simulink model "ARO40506DOF_2020a_2025_LAT"  (R2025b)
settings: Solver=VariableStepAuto  StartTime=0.0  StopTime=10.0  RelTol=1e-3
values from neighbouring files (symbols this model uses):
  Clbeta = -0.095    [Sim6DOF_Init.m]
  CldA = 0.014    [Sim6DOF_Init.m]
  CldR = 0.005    [Sim6DOF_Init.m]
  Cnbeta = 0.210    (= 0.21)    [Sim6DOF_Init.m]
  CndA = -0.0028    [Sim6DOF_Init.m]
  CndR = -0.095    [Sim6DOF_Init.m]
  Cybeta = -0.90    (= -0.9)    [Sim6DOF_Init.m]
  CydA = 0.0    (= 0)    [Sim6DOF_Init.m]
  CydR = 0.60    (= 0.6)    [Sim6DOF_Init.m]
  D2R = pi/180    (= 0.0174532925199)    [Sim6DOF_Init.m]
  q0 = 0    [Sim6DOF_Init.m]
  Span = 212.5    [Sim6DOF_Init.m]
  Sref = 4702    [Sim6DOF_Init.m]
  StabTrimPos = 5.5    [Sim6DOF_Init.m]
undefined symbols (not defined in the file or in its folder): Q
libraries: aerolibactuator x2
settings Model: Creator=Rainman  LastModifiedBy=Jordan Baylos
settings SolverCC: AlgebraicLoopSolver=TrustRegion
settings RTWCC: GPUComputeCapability=3.5

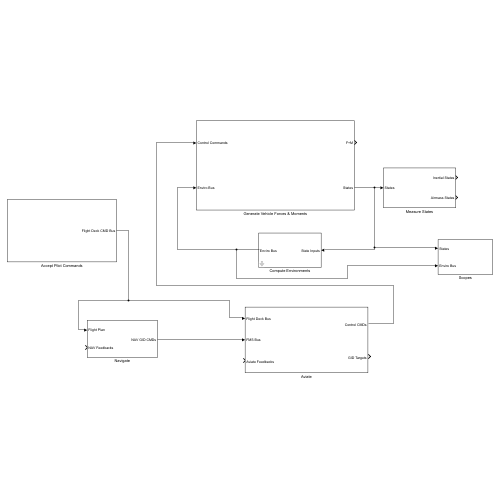
[thumbnail: Simulink's stored preview of the top-level diagram]
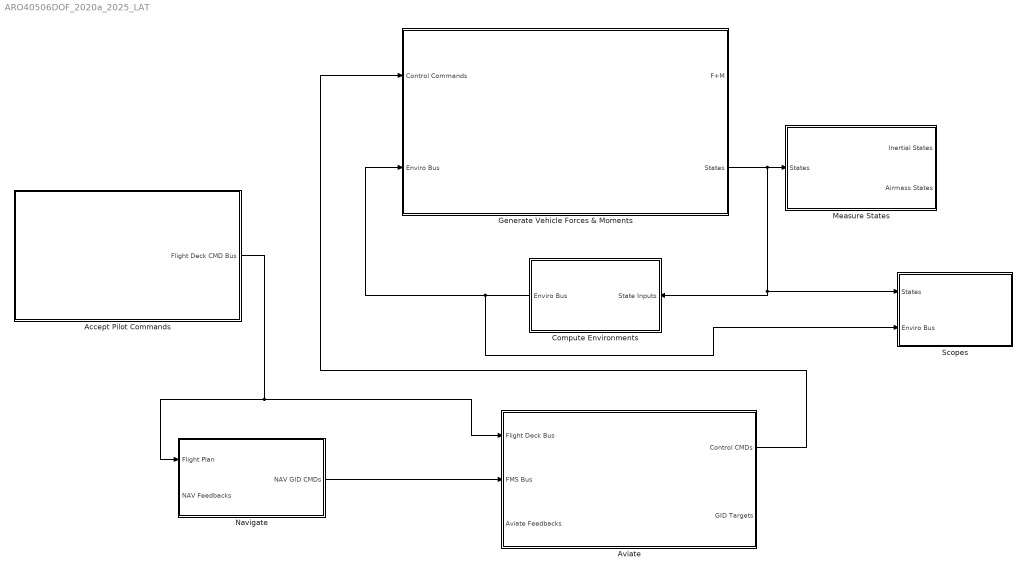
== system ARO40506DOF_2020a_2025_LAT ==
  Accept Pilot Commands : Subsystem
  Aviate : Subsystem
  Compute Environments : Subsystem
  Generate Vehicle Forces & Moments : Subsystem
  Measure States : Subsystem
  Navigate : Subsystem
  Scopes : Subsystem
  wires:
  Navigate/1(NAV GID CMDs) -> Aviate/2(FMS Bus)
  Aviate/1(Control CMDs) -> Generate Vehicle Forces & Moments/1(Control Commands)
  Accept Pilot Commands/1(Flight Deck CMD Bus) -> Navigate/1(Flight Plan), Aviate/1(Flight Deck Bus)
  Generate Vehicle Forces & Moments/2(States) -> Compute Environments/1(State Inputs), Scopes/1(States), Measure States/1(States)
  Compute Environments/1(Enviro Bus) -> Scopes/2(Enviro Bus), Generate Vehicle Forces & Moments/2(Enviro Bus)

== system ARO40506DOF_2020a_2025_LAT/Accept Pilot Commands ==
  Accept Control CMDs : Subsystem
  Accept Flight Plan CMDs : Subsystem
  Accept Guidance CMDs : Subsystem
  FLTDeck OUT : BusCreator  Inputs=3
  Flight Deck CMD Bus : Outport
  wires:
  FLTDeck OUT/1 -> Flight Deck CMD Bus/1
  Accept Flight Plan CMDs/1(Flight Plan) -> FLTDeck OUT/1  "Flight Plan"
  Accept Guidance CMDs/1(GID CMDs) -> FLTDeck OUT/2  "GID MCP CMDs"
  Accept Control CMDs/1(CTL CMDs) -> FLTDeck OUT/3  "Inceptor CMDs"

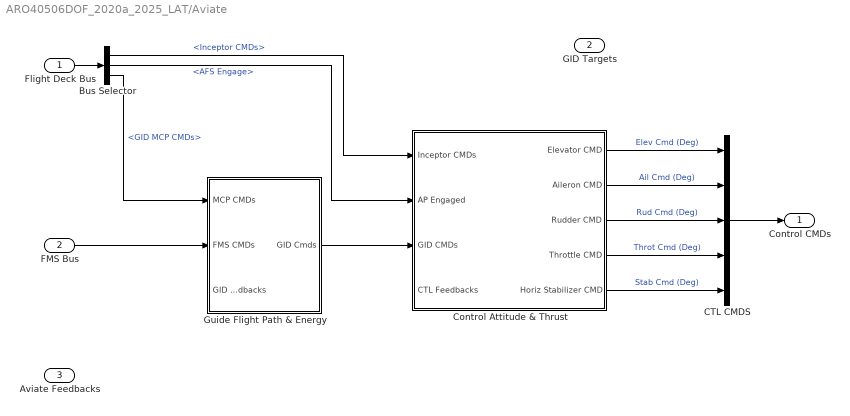
== system ARO40506DOF_2020a_2025_LAT/Aviate ==
  Flight Deck Bus : Inport
  FMS Bus : Inport  Port=2
  Aviate Feedbacks : Inport  Port=3
  Bus Selector : BusSelector  OutputSignals=Inceptor CMDs,GID MCP CMDs.AFS Engage,GID MCP CMDs
  CTL CMDS : BusCreator  Inputs=5
  Control Attitude & Thrust : Subsystem
  Guide Flight Path & Energy : Subsystem
  Control CMDs : Outport
  GID Targets : Outport  Port=2
  wires:
  CTL CMDS/1 -> Control CMDs/1
  Control Attitude & Thrust/1(Elevator CMD) -> CTL CMDS/1  "Elev Cmd (Deg)"
  Control Attitude & Thrust/2(Aileron CMD) -> CTL CMDS/2  "Ail Cmd (Deg)"
  Control Attitude & Thrust/3(Rudder CMD) -> CTL CMDS/3  "Rud Cmd (Deg)"
  Control Attitude & Thrust/4(Throttle CMD) -> CTL CMDS/4  "Throt Cmd (Deg)"
  FMS Bus/1 -> Guide Flight Path & Energy/2(FMS CMDs)
  Flight Deck Bus/1 -> Bus Selector/1
  Bus Selector/1 -> Control Attitude & Thrust/1(Inceptor CMDs)  "<Inceptor CMDs>"
  Bus Selector/3 -> Guide Flight Path & Energy/1(MCP CMDs)  "<GID MCP CMDs>"
  Control Attitude & Thrust/5(Horiz Stabilizer CMD) -> CTL CMDS/5  "Stab Cmd (Deg)"
  Guide Flight Path & Energy/1(GID Cmds) -> Control Attitude & Thrust/3(GID CMDs)
  Bus Selector/2 -> Control Attitude & Thrust/2(AP Engaged)  "<AFS Engage>"

== system ARO40506DOF_2020a_2025_LAT/Compute Environments ==
  State Inputs : Inport
  Environments : BusCreator  Inputs=8
  Enviro Bus : Outport
  wires:
  Environments/1 -> Enviro Bus/1
  ? -> Environments/5  "Q (Lb/Ft^2)"
  ? -> Environments/2  "Mach"
  ? -> Environments/4  "Density (Slug/Ft^3)"
  ? -> Environments/6  "Reynold's Num"
  ? -> Environments/3  "Altitude (Ft)"
  ? -> Environments/1  "Airspeed (Ft/Sec)"
  ? -> Environments/7  "Alpha (Deg)"
  ? -> Environments/8  "Beta (Deg)"

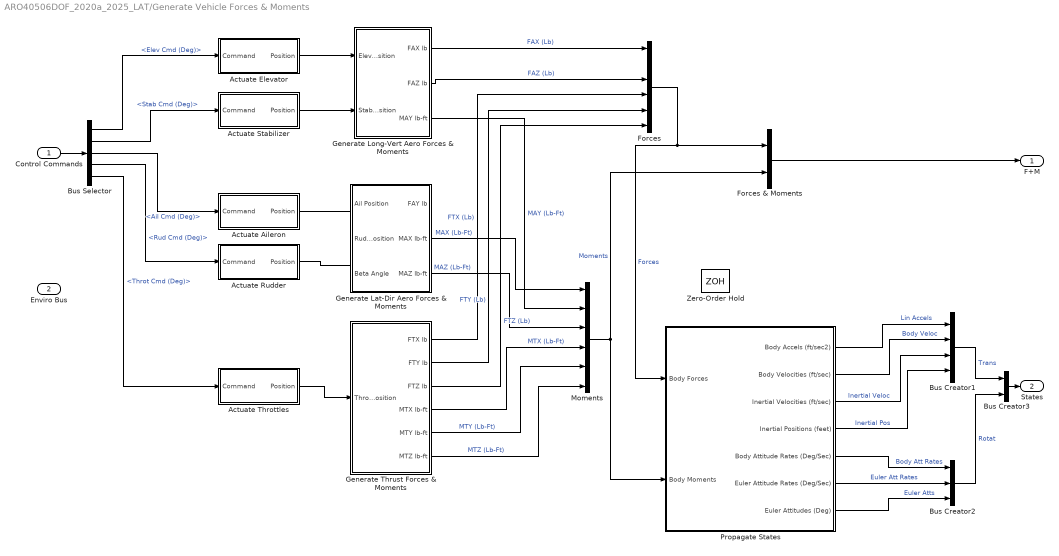
== system ARO40506DOF_2020a_2025_LAT/Generate Vehicle Forces & Moments ==
  Control Commands : Inport
  Enviro Bus : Inport  Port=2
  Actuate Aileron : Subsystem
  Actuate Elevator : Subsystem
  Actuate Rudder : Subsystem
  Actuate Stabilizer : Subsystem
  Actuate Throttles : Subsystem
  Bus Creator1 : BusCreator  Inputs=4
  Bus Creator2 : BusCreator  Inputs=3
  Bus Creator3 : BusCreator  Inputs=2
  Bus Selector : BusSelector  OutputSignals=Elev Cmd (Deg),Stab Cmd (Deg),Ail Cmd (Deg),Rud Cmd (Deg),Throt Cmd (Deg)
  Forces : BusCreator  Inputs=6
  Forces & Moments : BusCreator  Inputs=2
  Generate Lat-Dir Aero Forces & Moments : Subsystem
  Generate Long-Vert Aero Forces & Moments : Subsystem
  Generate Thrust Forces & Moments : Subsystem
  Moments : BusCreator  Inputs=6
  Propagate States : Subsystem
  Zero-Order Hold : ZeroOrderHold  SampleTime=-1
  F+M : Outport
  States : Outport  Port=2
  wires:
  Forces & Moments/1 -> F+M/1
  Bus Creator1/1 -> Bus Creator3/1  "Trans"
  Bus Creator2/1 -> Bus Creator3/2  "Rotat"
  Bus Creator3/1 -> States/1
  Propagate States/1(Body Accels (ft/sec2)) -> Bus Creator1/1  "Lin Accels"
  Propagate States/2(Body Velocities (ft/sec)) -> Bus Creator1/2  "Body Veloc"
  Propagate States/3(Inertial Velocities (ft/sec)) -> Bus Creator1/3  "Inertial Veloc"
  Propagate States/4(Inertial Positions (feet)) -> Bus Creator1/4  "Inertial Pos"
  Propagate States/5(Body Attitude Rates (Deg/Sec)) -> Bus Creator2/1  "Body Att Rates"
  Propagate States/6(Euler Attitude Rates (Deg/Sec)) -> Bus Creator2/2  "Euler Att Rates"
  Propagate States/7(Euler Attitudes (Deg)) -> Bus Creator2/3  "Euler Atts"
  Generate Long-Vert Aero Forces & Moments/1(FAX lb) -> Forces/1  "FAX (Lb)"
  Generate Long-Vert Aero Forces & Moments/2(FAZ lb) -> Forces/3  "FAZ (Lb)"
  ? -> Forces/2  "FAY (Lb)"
  Generate Lat-Dir Aero Forces & Moments/2(MAX lb-ft) -> Moments/1  "MAX (Lb-Ft)"
  Generate Long-Vert Aero Forces & Moments/3(MAY lb-ft) -> Moments/2  "MAY (Lb-Ft)"
  Generate Lat-Dir Aero Forces & Moments/3(MAZ lb-ft) -> Moments/3  "MAZ (Lb-Ft)"
  Forces/1 -> Propagate States/1(Body Forces), Forces & Moments/1  "Forces"
  Moments/1 -> Forces & Moments/2, Propagate States/2(Body Moments)  "Moments"
  Control Commands/1 -> Bus Selector/1
  Bus Selector/1 -> Actuate Elevator/1(Command)  "<Elev Cmd (Deg)>"
  Actuate Elevator/1(Position) -> Generate Long-Vert Aero Forces & Moments/1(Elev Position)
  Actuate Aileron/1(Position) -> ?
  Actuate Rudder/1(Position) -> ?
  Bus Selector/4 -> Actuate Rudder/1(Command)  "<Rud Cmd (Deg)>"
  Bus Selector/3 -> Actuate Aileron/1(Command)  "<Ail Cmd (Deg)>"
  Actuate Throttles/1(Position) -> Generate Thrust Forces & Moments/1(Throt Position)
  Bus Selector/5 -> Actuate Throttles/1(Command)  "<Throt Cmd (Deg)>"
  Bus Selector/2 -> Actuate Stabilizer/1(Command)  "<Stab Cmd (Deg)>"
  Actuate Stabilizer/1(Position) -> Generate Long-Vert Aero Forces & Moments/2(Stab Position)
  Generate Thrust Forces & Moments/1(FTX lb) -> Forces/4  "FTX (Lb)"
  Generate Thrust Forces & Moments/2(FTY lb) -> Forces/5  "FTY (Lb)"
  Generate Thrust Forces & Moments/3(FTZ lb) -> Forces/6  "FTZ (Lb)"
  Generate Thrust Forces & Moments/4(MTX lb-ft) -> Moments/4  "MTX (Lb-Ft)"
  Generate Thrust Forces & Moments/5(MTY lb-ft) -> Moments/5  "MTY (Lb-Ft)"
  Generate Thrust Forces & Moments/6(MTZ lb-ft) -> Moments/6  "MTZ (Lb-Ft)"

== system ARO40506DOF_2020a_2025_LAT/Measure States ==
  States : Inport
  Inertial States : Outport
  Airmass States : Outport  Port=2

== system ARO40506DOF_2020a_2025_LAT/Navigate ==
  Flight Plan : Inport
  NAV Feedbacks : Inport  Port=2
  Bus Creator : BusCreator  Inputs=4
  NAV GID CMDs : Outport
  wires:
  Bus Creator/1 -> NAV GID CMDs/1  "FMS GID Cmds"
  ? -> Bus Creator/1  "FMS ALT Target"
  ? -> Bus Creator/2  "FMS VS Target"
  ? -> Bus Creator/3  "FMS HDG Target"
  ? -> Bus Creator/4  "FMS SPD Target"

== system ARO40506DOF_2020a_2025_LAT/Scopes ==
  States : Inport
  Enviro Bus : Inport  Port=2
  Bus Selector : BusSelector  OutputSignals=Alpha (Deg),Airspeed (Ft/Sec),Altitude (Ft),Beta (Deg)
  Bus Selector1 : BusSelector  OutputSignals=Rotat.Euler Atts.Pitch Attitude (Deg),Rotat.Euler Att Rates.Pitch Att Rate (Deg/Sec),Rotat.Euler Atts.Roll Attitude (Deg),Rotat.Euler Att Rates.Roll Att Rate (Deg/Sec),Rotat.Euler Atts.Heading (Deg)
  Lat-Dir : Scope  NumInputPorts=7
  Long-Vert : Scope  NumInputPorts=7
  wires:
  States/1 -> Bus Selector1/1
  Enviro Bus/1 -> Bus Selector/1
  Bus Selector/3 -> Long-Vert/3  "<Altitude (Ft)>"
  Bus Selector1/1 -> Long-Vert/1  "<Pitch Attitude (Deg)>"
  Bus Selector1/2 -> Long-Vert/2  "<Pitch Att Rate (Deg/Sec)>"
  Bus Selector/2 -> Long-Vert/7  "<Airspeed (Ft/Sec)>"
  Bus Selector1/3 -> Lat-Dir/1  "<Roll Attitude (Deg)>"
  Bus Selector1/5 -> Lat-Dir/3  "<Heading (Deg)>"
  Bus Selector/1 -> Long-Vert/4  "<Alpha (Deg)>"
  Bus Selector/4 -> Lat-Dir/4  "<Beta (Deg)>"
  Bus Selector1/4 -> Lat-Dir/2  "<Roll Att Rate (Deg/Sec)>"

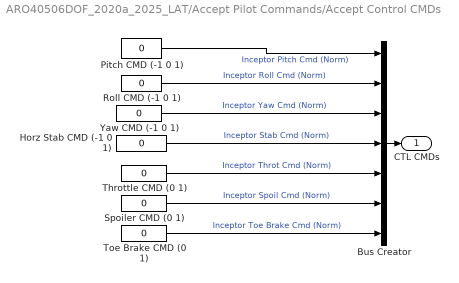
== system ARO40506DOF_2020a_2025_LAT/Accept Pilot Commands/Accept Control CMDs ==
  Bus Creator : BusCreator  Inputs=7
  Horz Stab CMD (-1 0 1) : Constant  Value=0
  Pitch CMD (-1 0 1) : Constant  Value=0
  Roll CMD (-1 0 1) : Constant  Value=0
  Spoiler CMD (0 1) : Constant  Value=0
  Throttle CMD (0 1) : Constant  Value=0
  Toe Brake CMD (0 1) : Constant  Value=0
  Yaw CMD (-1 0 1) : Constant  Value=0
  CTL CMDs : Outport
  wires:
  Pitch CMD (-1 0 1)/1 -> Bus Creator/1  "Inceptor Pitch Cmd (Norm)"
  Roll CMD (-1 0 1)/1 -> Bus Creator/2  "Inceptor Roll Cmd (Norm)"
  Yaw CMD (-1 0 1)/1 -> Bus Creator/3  "Inceptor Yaw Cmd (Norm)"
  Throttle CMD (0 1)/1 -> Bus Creator/5  "Inceptor Throt Cmd (Norm)"
  Spoiler CMD (0 1)/1 -> Bus Creator/6  "Inceptor Spoil Cmd (Norm)"
  Toe Brake CMD (0 1)/1 -> Bus Creator/7  "Inceptor Toe Brake Cmd (Norm)"
  Horz Stab CMD (-1 0 1)/1 -> Bus Creator/4  "Inceptor Stab Cmd (Norm)"
  Bus Creator/1 -> CTL CMDs/1

== system ARO40506DOF_2020a_2025_LAT/Accept Pilot Commands/Accept Flight Plan CMDs ==
  Flight Plan : Outport

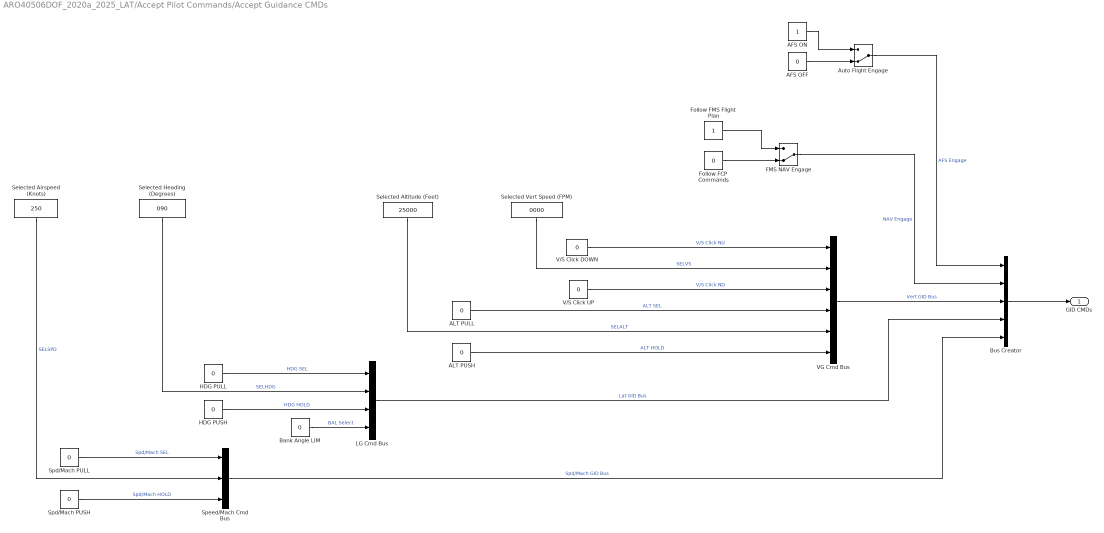
== system ARO40506DOF_2020a_2025_LAT/Accept Pilot Commands/Accept Guidance CMDs ==
  AFS OFF : Constant  Value=0
  AFS ON : Constant
  ALT PULL : Constant  Value=0
  ALT PUSH : Constant  Value=0
  Auto Flight Engage : ManualSwitch  CurrentSetting=0
  Bank Angle LIM : Constant  Value=0
  Bus Creator : BusCreator  Inputs=5
  FMS NAV Engage : ManualSwitch  CurrentSetting=0
  Follow FCP Commands : Constant  Value=0
  Follow FMS Flight Plan : Constant
  HDG PULL : Constant  Value=0
  HDG PUSH : Constant  Value=0
  LG Cmd Bus : BusCreator  Inputs=4
  Selected Airspeed (Knots) : Constant  Value=250
  Selected Altitude (Feet) : Constant  Value=25000
  Selected Heading (Degrees) : Constant  Value=090
  Selected Vert Speed (FPM) : Constant  Value=0000
  Spd/Mach PULL : Constant  Value=0
  Spd/Mach PUSH : Constant  Value=0
  Speed/Mach Cmd Bus : BusCreator  Inputs=3
  V/S Click DOWN : Constant  Value=0
  V/S Click UP : Constant  Value=0
  VG Cmd Bus : BusCreator  Inputs=6
  GID CMDs : Outport
  wires:
  Bus Creator/1 -> GID CMDs/1
  VG Cmd Bus/1 -> Bus Creator/3  "Vert GID Bus"
  LG Cmd Bus/1 -> Bus Creator/4  "Lat GID Bus"
  Speed/Mach Cmd Bus/1 -> Bus Creator/5  "Spd/Mach GID Bus"
  Selected Altitude (Feet)/1 -> VG Cmd Bus/5  "SELALT"
  Selected Vert Speed (FPM)/1 -> VG Cmd Bus/2  "SELVS"
  Selected Heading (Degrees)/1 -> LG Cmd Bus/2  "SELHDG"
  Selected Airspeed (Knots)/1 -> Speed/Mach Cmd Bus/2  "SELSPD"
  Auto Flight Engage/1 -> Bus Creator/1  "AFS Engage"
  AFS ON/1 -> Auto Flight Engage/1
  AFS OFF/1 -> Auto Flight Engage/2
  Follow FMS Flight Plan/1 -> FMS NAV Engage/1
  Follow FCP Commands/1 -> FMS NAV Engage/2
  FMS NAV Engage/1 -> Bus Creator/2  "NAV Engage"
  Bank Angle LIM/1 -> LG Cmd Bus/4  "BAL Select"
  HDG PULL/1 -> LG Cmd Bus/1  "HDG SEL"
  HDG PUSH/1 -> LG Cmd Bus/3  "HDG HOLD"
  Spd/Mach PUSH/1 -> Speed/Mach Cmd Bus/3  "Spd/Mach HOLD"
  Spd/Mach PULL/1 -> Speed/Mach Cmd Bus/1  "Spd/Mach SEL"
  V/S Click DOWN/1 -> VG Cmd Bus/1  "V/S Click NU"
  V/S Click UP/1 -> VG Cmd Bus/3  "V/S Click ND"
  ALT PULL/1 -> VG Cmd Bus/4  "ALT SEL"
  ALT PUSH/1 -> VG Cmd Bus/6  "ALT HOLD"

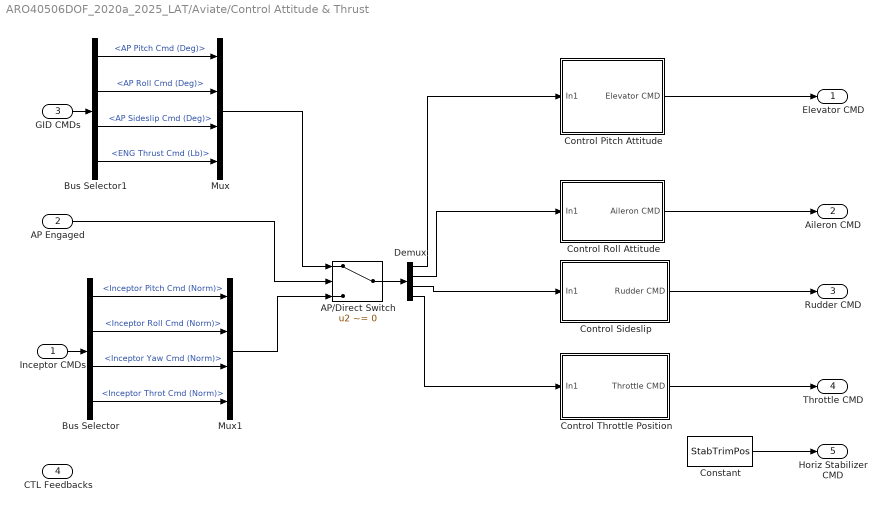
== system ARO40506DOF_2020a_2025_LAT/Aviate/Control Attitude & Thrust ==
  Inceptor CMDs : Inport
  AP Engaged : Inport  Port=2
  GID CMDs : Inport  Port=3
  CTL Feedbacks : Inport  Port=4
  AP/Direct Switch : Switch  Criteria=u2 ~= 0  SaturateOnIntegerOverflow=off  InputSameDT=off
  Bus Selector : BusSelector  OutputSignals=Inceptor Pitch Cmd (Norm),Inceptor Roll Cmd (Norm),Inceptor Yaw Cmd (Norm),Inceptor Throt Cmd (Norm)
  Bus Selector1 : BusSelector  OutputSignals=AP Pitch Cmd (Deg),AP Roll Cmd (Deg),AP Sideslip Cmd (Deg),ENG Thrust Cmd (Lb)
  Constant : Constant  Value=StabTrimPos
  Control Pitch Attitude : Subsystem
  Control Roll Attitude : Subsystem
  Control Sideslip : Subsystem
  Control Throttle Position : Subsystem
  Demux : Demux
  Mux : Mux
  Mux1 : Mux
  Elevator CMD : Outport
  Aileron CMD : Outport  Port=2
  Rudder CMD : Outport  Port=3
  Throttle CMD : Outport  Port=4
  Horiz Stabilizer CMD : Outport  Port=5
  wires:
  Inceptor CMDs/1 -> Bus Selector/1
  Bus Selector/1 -> Mux1/1  "<Inceptor Pitch Cmd (Norm)>"
  GID CMDs/1 -> Bus Selector1/1
  Bus Selector1/4 -> Mux/4  "<ENG Thrust Cmd (Lb)>"
  Bus Selector/2 -> Mux1/2  "<Inceptor Roll Cmd (Norm)>"
  Bus Selector1/2 -> Mux/2  "<AP Roll Cmd (Deg)>"
  Bus Selector1/1 -> Mux/1  "<AP Pitch Cmd (Deg)>"
  Bus Selector1/3 -> Mux/3  "<AP Sideslip Cmd (Deg)>"
  Bus Selector/3 -> Mux1/3  "<Inceptor Yaw Cmd (Norm)>"
  Bus Selector/4 -> Mux1/4  "<Inceptor Throt Cmd (Norm)>"
  Mux/1 -> AP/Direct Switch/1
  AP Engaged/1 -> AP/Direct Switch/2
  Mux1/1 -> AP/Direct Switch/3
  AP/Direct Switch/1 -> Demux/1
  Demux/1 -> Control Pitch Attitude/1(In1)
  Demux/2 -> Control Roll Attitude/1(In1)
  Demux/3 -> Control Sideslip/1(In1)
  Demux/4 -> Control Throttle Position/1(In1)
  Control Pitch Attitude/1(Elevator CMD) -> Elevator CMD/1
  Control Roll Attitude/1(Aileron CMD) -> Aileron CMD/1
  Control Throttle Position/1(Throttle CMD) -> Throttle CMD/1
  Control Sideslip/1(Rudder CMD) -> Rudder CMD/1
  Constant/1 -> Horiz Stabilizer CMD/1

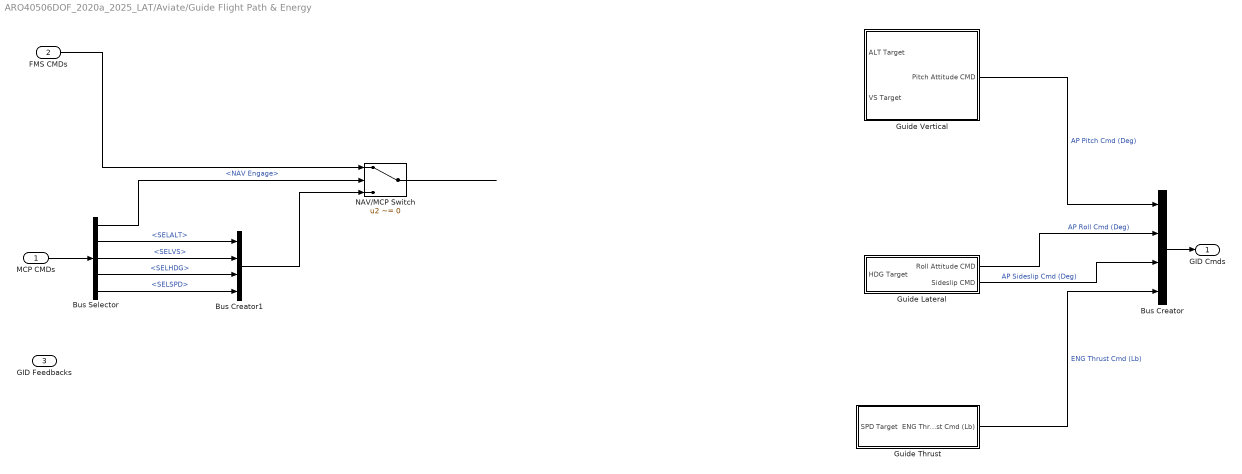
== system ARO40506DOF_2020a_2025_LAT/Aviate/Guide Flight Path & Energy ==
  MCP CMDs : Inport
  FMS CMDs : Inport  Port=2
  GID Feedbacks : Inport  Port=3
  Bus Creator : BusCreator  Inputs=4
  Bus Creator1 : BusCreator  Inputs=4
  Bus Selector : BusSelector  OutputSignals=NAV Engage,Vert GID Bus.SELALT,Vert GID Bus.SELVS,Lat GID Bus.SELHDG,Spd/Mach GID Bus.SELSPD
  Guide Lateral : Subsystem
  Guide Thrust : Subsystem
  Guide Vertical : Subsystem
  NAV/MCP Switch : Switch  Criteria=u2 ~= 0  SaturateOnIntegerOverflow=off  InputSameDT=off
  GID Cmds : Outport
  wires:
  Guide Vertical/1(Pitch Attitude CMD) -> Bus Creator/1  "AP Pitch Cmd (Deg)"
  Guide Lateral/1(Roll Attitude CMD) -> Bus Creator/2  "AP Roll Cmd (Deg)"
  Guide Lateral/2(Sideslip CMD) -> Bus Creator/3  "AP Sideslip Cmd (Deg)"
  Guide Thrust/1(ENG Thrust Cmd (Lb)) -> Bus Creator/4  "ENG Thrust Cmd (Lb)"
  Bus Creator/1 -> GID Cmds/1
  MCP CMDs/1 -> Bus Selector/1
  Bus Selector/1 -> NAV/MCP Switch/2  "<NAV Engage>"
  Bus Selector/2 -> Bus Creator1/1  "<SELALT>"
  Bus Selector/3 -> Bus Creator1/2  "<SELVS>"
  Bus Selector/4 -> Bus Creator1/3  "<SELHDG>"
  Bus Selector/5 -> Bus Creator1/4  "<SELSPD>"
  FMS CMDs/1 -> NAV/MCP Switch/1
  Bus Creator1/1 -> NAV/MCP Switch/3
  NAV/MCP Switch/1 -> ?

== system ARO40506DOF_2020a_2025_LAT/Generate Vehicle Forces & Moments/Actuate Aileron ==
  Command : Inport
  Actuator 1st Order Model : TransferFcn  Denominator=[0.5 1]
  Position Limit : Saturate  UpperLimit=30  LowerLimit=-30
  Position : Outport
  wires:
  Command/1 -> Position Limit/1
  Position Limit/1 -> Actuator 1st Order Model/1
  Actuator 1st Order Model/1 -> Position/1

== system ARO40506DOF_2020a_2025_LAT/Generate Vehicle Forces & Moments/Actuate Elevator ==
  Command : Inport
  Actuator 1st Order Model : TransferFcn  Denominator=[0.5 1]
  Position Limit : Saturate  UpperLimit=30  LowerLimit=-30
  Position : Outport
  wires:
  Command/1 -> Position Limit/1
  Position Limit/1 -> Actuator 1st Order Model/1
  Actuator 1st Order Model/1 -> Position/1

== system ARO40506DOF_2020a_2025_LAT/Generate Vehicle Forces & Moments/Actuate Rudder ==
  Command : Inport
  Actuator 1st Order Model : TransferFcn  Denominator=[0.5 1]
  Position Limit : Saturate  UpperLimit=30  LowerLimit=-30
  Position : Outport
  wires:
  Command/1 -> Position Limit/1
  Position Limit/1 -> Actuator 1st Order Model/1
  Actuator 1st Order Model/1 -> Position/1

== system ARO40506DOF_2020a_2025_LAT/Generate Vehicle Forces & Moments/Actuate Stabilizer ==
  Command : Inport
  Position Limit : Saturate  UpperLimit=15  LowerLimit=-5
  Stabilizer Actuator : aerolibactuator/Linear Second-Order Actuator  wn_fin=0.3  z_fin=1.0  fin_act_0=0  fin_act_vel=0
  Position : Outport
  wires:
  Command/1 -> Position Limit/1
  Position Limit/1 -> Stabilizer Actuator/1
  Stabilizer Actuator/1 -> Position/1

== system ARO40506DOF_2020a_2025_LAT/Generate Vehicle Forces & Moments/Actuate Throttles ==
  Command : Inport
  Position Limit : Saturate  UpperLimit=100  LowerLimit=0
  Throttle Actuator : aerolibactuator/Linear Second-Order Actuator  wn_fin=1  z_fin=1.0  fin_act_0=0  fin_act_vel=0
  Position : Outport
  wires:
  Command/1 -> Position Limit/1
  Position Limit/1 -> Throttle Actuator/1
  Throttle Actuator/1 -> Position/1

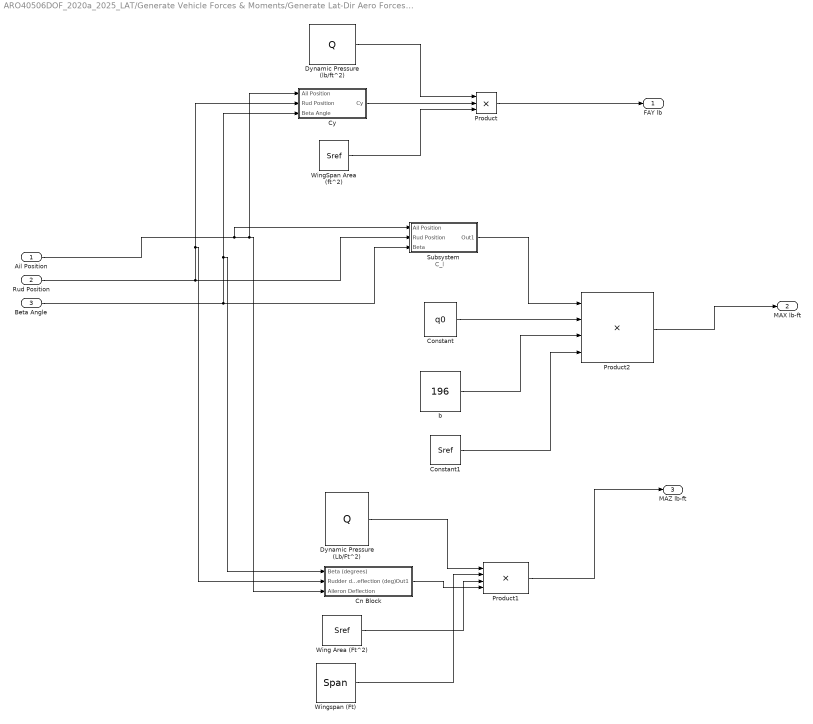
== system ARO40506DOF_2020a_2025_LAT/Generate Vehicle Forces & Moments/Generate Lat-Dir Aero Forces & Moments ==
  note: C_l
  Ail Position : Inport
  Rud Position : Inport  Port=2
  Beta Angle : Inport  Port=3
  Cn Block : Subsystem
  Constant : Constant  Value=q0
  Constant1 : Constant  Value=Sref
  Cy : Subsystem
  Dynamic Pressure (Lb/Ft^2) : Constant  Value=Q
  Dynamic Pressure (lb/ft^2) : Constant  Value=Q
  Product : Product  Inputs=3
  Product1 : Product  Inputs=****
  Product2 : Product  Inputs=4
  Subsystem : Subsystem
  Wing Area (Ft^2) : Constant  Value=Sref
  WingSpan Area (ft^2) : Constant  Value=Sref
  Wingspan (Ft) : Constant  Value=Span
  b : Constant  Value=196
  FAY lb : Outport
  MAX lb-ft : Outport  Port=2
  MAZ lb-ft : Outport  Port=3
  wires:
  Dynamic Pressure (lb/ft^2)/1 -> Product/1
  Product/1 -> FAY lb/1
  WingSpan Area (ft^2)/1 -> Product/3
  Cy/1(Cy) -> Product/2
  Product1/1 -> MAZ lb-ft/1
  Wing Area (Ft^2)/1 -> Product1/3
  Cn Block/1(Out1) -> Product1/4
  Wingspan (Ft)/1 -> Product1/2
  Dynamic Pressure (Lb/Ft^2)/1 -> Product1/1
  b/1 -> Product2/3
  Product2/1 -> MAX lb-ft/1
  Constant/1 -> Product2/2
  Beta Angle/1 -> Subsystem/3(Beta), Cn Block/1(Beta (degrees)), Cy/3(Beta Angle)
  Ail Position/1 -> Subsystem/1(Ail Position), Cn Block/3(Aileron Deflection), Cy/1(Ail Position)
  Constant1/1 -> Product2/4
  Rud Position/1 -> Subsystem/2(Rud Position), Cn Block/2(Rudder deflection (deg)), Cy/2(Rud Position)
  Subsystem/1(Out1) -> Product2/1

== system ARO40506DOF_2020a_2025_LAT/Generate Vehicle Forces & Moments/Generate Long-Vert Aero Forces & Moments ==
  Elev Position : Inport
  Stab Position : Inport  Port=2
  FAX lb : Outport
  FAZ lb : Outport  Port=2
  MAY lb-ft : Outport  Port=3

== system ARO40506DOF_2020a_2025_LAT/Generate Vehicle Forces & Moments/Generate Thrust Forces & Moments ==
  Throt Position : Inport
  FTX lb : Outport
  FTY lb : Outport  Port=2
  FTZ lb : Outport  Port=3
  MTX lb-ft : Outport  Port=4
  MTY lb-ft : Outport  Port=5
  MTZ lb-ft : Outport  Port=6

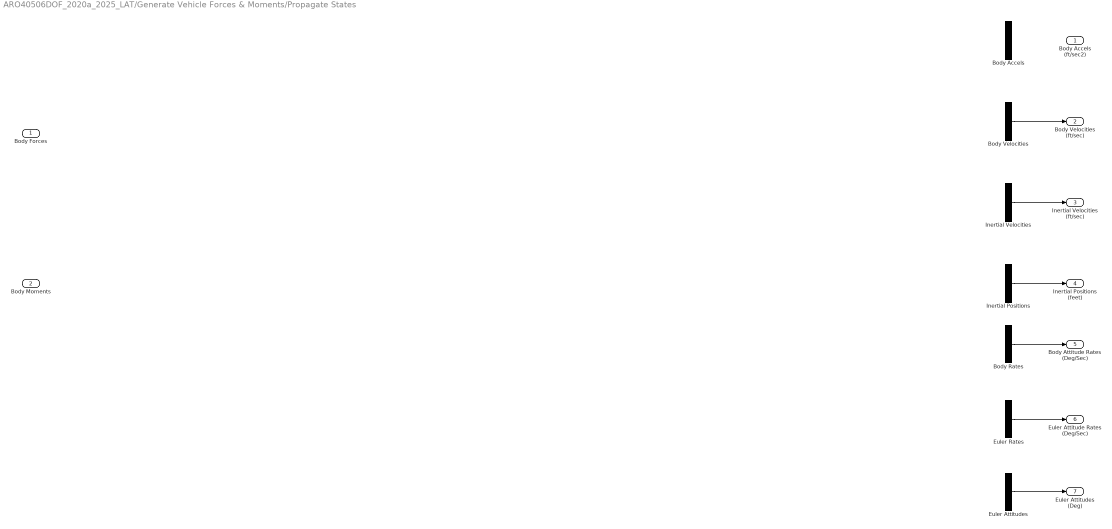
== system ARO40506DOF_2020a_2025_LAT/Generate Vehicle Forces & Moments/Propagate States ==
  Body Forces : Inport
  Body Moments : Inport  Port=2
  Body Accels : BusCreator  Inputs=3
  Body Rates : BusCreator  Inputs=3
  Body Velocities : BusCreator  Inputs=3
  Euler Attitudes : BusCreator  Inputs=3
  Euler Rates : BusCreator  Inputs=3
  Inertial Positions : BusCreator  Inputs=3
  Inertial Velocities : BusCreator  Inputs=3
  Body Accels (ft/sec2) : Outport
  Body Velocities (ft/sec) : Outport  Port=2
  Inertial Velocities (ft/sec) : Outport  Port=3
  Inertial Positions (feet) : Outport  Port=4
  Body Attitude Rates (Deg/Sec) : Outport  Port=5
  Euler Attitude Rates (Deg/Sec) : Outport  Port=6
  Euler Attitudes (Deg) : Outport  Port=7
  wires:
  Euler Attitudes/1 -> Euler Attitudes (Deg)/1
  ? -> Euler Attitudes/3  "Heading (Deg)"
  ? -> Euler Attitudes/2  "Roll Attitude (Deg)"
  ? -> Euler Attitudes/1  "Pitch Attitude (Deg)"
  Euler Rates/1 -> Euler Attitude Rates (Deg/Sec)/1
  Body Rates/1 -> Body Attitude Rates (Deg/Sec)/1
  Inertial Positions/1 -> Inertial Positions (feet)/1
  Inertial Velocities/1 -> Inertial Velocities (ft/sec)/1
  Body Velocities/1 -> Body Velocities (ft/sec)/1
  ? -> Body Accels/1  "Longitudinal Accel (Ft/Sec^2)"
  ? -> Body Accels/2  "Lateral Accel (Ft/Sec^2)"
  ? -> Body Accels/3  "Vertical Accel (Ft/Sec^2)"
  ? -> Euler Rates/1  "Pitch Att Rate (Deg/Sec)"
  ? -> Euler Rates/3  "Heading Att Rate (Deg/Sec)"
  ? -> Euler Rates/2  "Roll Att Rate (Deg/Sec)"
  ? -> Body Rates/1  "Pitch Rate (Deg/Sec)"
  ? -> Body Rates/3  "Yaw Rate (Deg/Sec)"
  ? -> Body Rates/2  "Roll Rate (Deg/Sec)"
  ? -> Inertial Positions/3  "Inertial Altitude (Feet)"
  ? -> Inertial Positions/1  "Latitude (Feet)"
  ? -> Inertial Positions/2  "Longitude (Feet)"
  ? -> Inertial Velocities/3  "Inertial Vertical Speed (Feet/Sec)"
  ? -> Inertial Velocities/1  "North-South Velocity (Feet/Sec)"
  ? -> Inertial Velocities/2  "East-West Velocity (Feet/Sec)"
  ? -> Body Velocities/3  "w (Feet/Sec)"
  ? -> Body Velocities/1  "u (Feet/Sec)"
  ? -> Body Velocities/2  "v (Feet/Sec)"

== system ARO40506DOF_2020a_2025_LAT/Aviate/Control Attitude & Thrust/Control Pitch Attitude ==
  In1 : Inport
  Elevator CMD : Outport
  wires:
  In1/1 -> Elevator CMD/1

== system ARO40506DOF_2020a_2025_LAT/Aviate/Control Attitude & Thrust/Control Roll Attitude ==
  In1 : Inport
  Aileron CMD : Outport
  wires:
  In1/1 -> Aileron CMD/1

== system ARO40506DOF_2020a_2025_LAT/Aviate/Control Attitude & Thrust/Control Sideslip ==
  In1 : Inport
  Rudder CMD : Outport
  wires:
  In1/1 -> Rudder CMD/1

== system ARO40506DOF_2020a_2025_LAT/Aviate/Control Attitude & Thrust/Control Throttle Position ==
  In1 : Inport
  Throttle CMD : Outport
  wires:
  In1/1 -> Throttle CMD/1

== system ARO40506DOF_2020a_2025_LAT/Aviate/Guide Flight Path & Energy/Guide Lateral ==
  HDG Target : Inport
  Roll Attitude CMD : Outport
  Sideslip CMD : Outport  Port=2

== system ARO40506DOF_2020a_2025_LAT/Aviate/Guide Flight Path & Energy/Guide Thrust ==
  SPD Target : Inport
  ENG Thrust Cmd (Lb) : Outport

== system ARO40506DOF_2020a_2025_LAT/Aviate/Guide Flight Path & Energy/Guide Vertical ==
  ALT Target : Inport
  VS Target : Inport  Port=2
  Pitch Attitude CMD : Outport

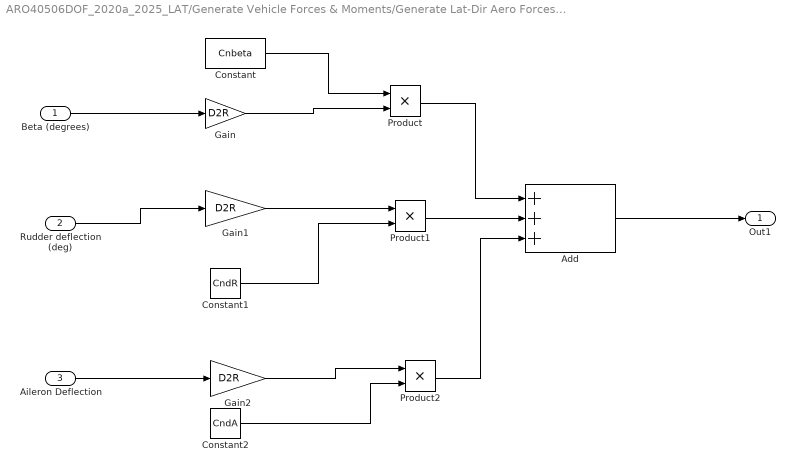
== system ARO40506DOF_2020a_2025_LAT/Generate Vehicle Forces & Moments/Generate Lat-Dir Aero Forces & Moments/Cn Block ==
  Beta (degrees) : Inport
  Rudder deflection (deg) : Inport  Port=2
  Aileron Deflection : Inport  Port=3
  Add : Sum  Inputs=+++
  Constant : Constant  Value=Cnbeta
  Constant1 : Constant  Value=CndR
  Constant2 : Constant  Value=CndA
  Gain : Gain  Gain=D2R
  Gain1 : Gain  Gain=D2R
  Gain2 : Gain  Gain=D2R
  Product : Product
  Product1 : Product
  Product2 : Product
  Out1 : Outport
  wires:
  Beta (degrees)/1 -> Gain/1
  Rudder deflection (deg)/1 -> Gain1/1
  Aileron Deflection/1 -> Gain2/1
  Constant/1 -> Product/1
  Gain/1 -> Product/2
  Constant1/1 -> Product1/2
  Gain1/1 -> Product1/1
  Gain2/1 -> Product2/1
  Constant2/1 -> Product2/2
  Product/1 -> Add/1
  Product1/1 -> Add/2
  Product2/1 -> Add/3
  Add/1 -> Out1/1

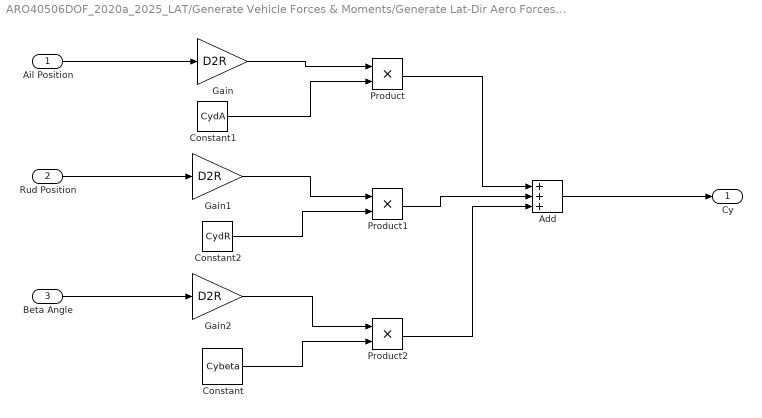
== system ARO40506DOF_2020a_2025_LAT/Generate Vehicle Forces & Moments/Generate Lat-Dir Aero Forces & Moments/Cy ==
  Ail Position : Inport
  Rud Position : Inport  Port=2
  Beta Angle : Inport  Port=3
  Add : Sum  Inputs=+++
  Constant : Constant  Value=Cybeta
  Constant1 : Constant  Value=CydA
  Constant2 : Constant  Value=CydR
  Gain : Gain  Gain=D2R
  Gain1 : Gain  Gain=D2R
  Gain2 : Gain  Gain=D2R
  Product : Product
  Product1 : Product
  Product2 : Product
  Cy : Outport
  wires:
  Ail Position/1 -> Gain/1
  Rud Position/1 -> Gain1/1
  Beta Angle/1 -> Gain2/1
  Gain/1 -> Product/1
  Constant1/1 -> Product/2
  Gain1/1 -> Product1/1
  Constant2/1 -> Product1/2
  Gain2/1 -> Product2/1
  Constant/1 -> Product2/2
  Product/1 -> Add/1
  Product1/1 -> Add/2
  Product2/1 -> Add/3
  Add/1 -> Cy/1

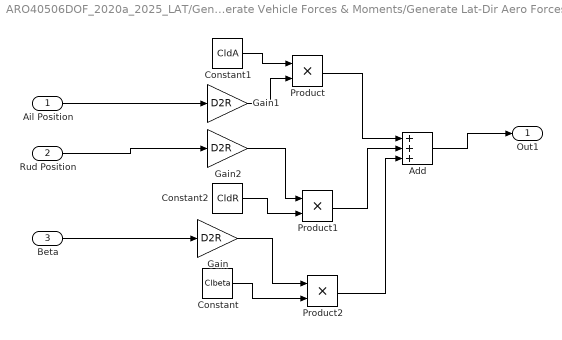
== system ARO40506DOF_2020a_2025_LAT/Generate Vehicle Forces & Moments/Generate Lat-Dir Aero Forces & Moments/Subsystem ==
  Ail Position : Inport
  Rud Position : Inport  Port=2
  Beta : Inport  Port=3
  Add : Sum  Inputs=+++
  Constant : Constant  Value=Clbeta
  Constant1 : Constant  Value=CldA
  Constant2 : Constant  Value=CldR
  Gain : Gain  Gain=D2R
  Gain1 : Gain  Gain=D2R
  Gain2 : Gain  Gain=D2R
  Product : Product
  Product1 : Product
  Product2 : Product
  Out1 : Outport
  wires:
  Beta/1 -> Gain/1
  Ail Position/1 -> Gain1/1
  Rud Position/1 -> Gain2/1
  Gain/1 -> Product2/1
  Constant/1 -> Product2/2
  Constant2/1 -> Product1/2
  Gain2/1 -> Product1/1
  Gain1/1 -> Product/2
  Constant1/1 -> Product/1
  Product/1 -> Add/1
  Product1/1 -> Add/2
  Product2/1 -> Add/3
  Add/1 -> Out1/1
